simulink model "samePIDmodelworkingdecoupler_customsignal"  (R2018a)
settings: Solver=VariableStepAuto  StartTime=0.0  StopTime=100  RelTol=1e-3
undefined symbols (not defined in the file): sigbuilder_block
libraries: simulink x2
settings Model: Creator=40292302  LastModifiedBy=40292302

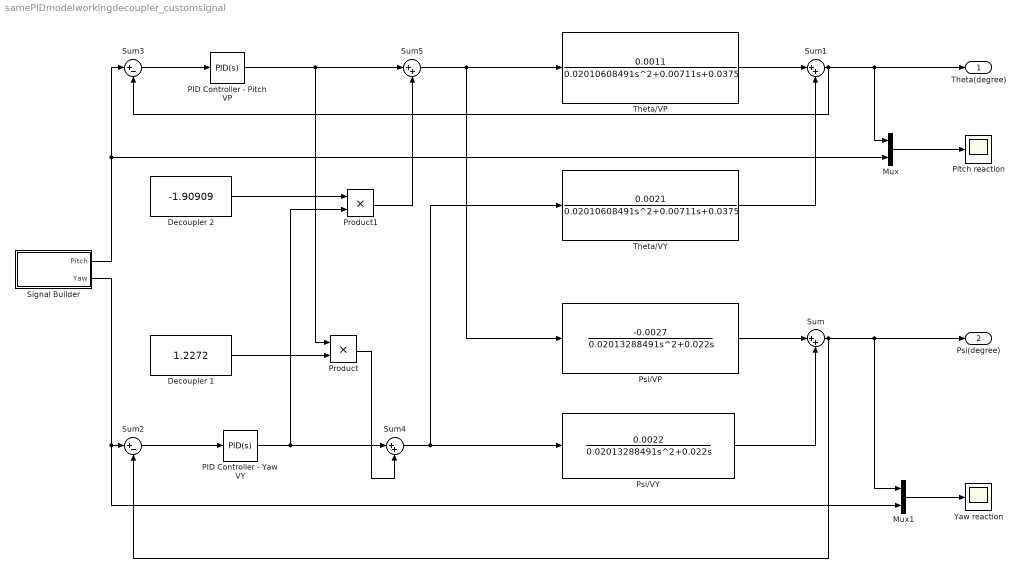
== system samePIDmodelworkingdecoupler_customsignal ==
  Decoupler 1 : Constant  Value=1.2272
  Decoupler 2 : Constant  Value=-1.90909
  Mux : Mux  Inputs=2
  Mux1 : Mux  Inputs=2
  PID Controller - Pitch VP : simulink/Continuous/PID Controller  Controller=PID  TimeDomain=Continuous-time  SampleTime=-1  IntegratorMethod=Forward Euler  FilterMethod=Forward Euler  Form=Parallel  UseFilter=on  ControllerParametersSource=internal  P=6813.01742872752  I=13170.6613633077  D=853.093750479044  N=251.511422827374  InitialConditionSource=internal  InitialConditionForIntegrator=0  InitialConditionForFilter=0  ExternalReset=none  LimitOutput=off  UpperSaturationLimit=inf  LowerSaturationLimit=-inf  LinearizeAsGain=on  AntiWindupMode=none  Kb=1  TrackingMode=off  Kt=1  PParamMin=[]  PParamMax=[]  IParamMin=[]  IParamMax=[]  DParamMin=[]  DParamMax=[]  NParamMin=[]  NParamMax=[]  KbParamMin=[]  KbParamMax=[]  KtParamMin=[]  KtParamMax=[]  POutMin=[]  POutMax=[]  IOutMin=[]  IOutMax=[]  DOutMin=[]  DOutMax=[]  NOutMin=[]  NOutMax=[]  KbOutMin=[]  KbOutMax=[]  KtOutMin=[]  KtOutMax=[]  IntegratorOutMin=[]  IntegratorOutMax=[]  FilterOutMin=[]  FilterOutMax=[]  SumOutMin=[]  SumOutMax=[]  SumI1OutMin=[]  SumI1OutMax=[]  SumI2OutMin=[]  SumI2OutMax=[]  SumI3OutMin=[]  SumI3OutMax=[]  SumDOutMin=[]  SumDOutMax=[]  SaturationOutMin=[]  SaturationOutMax=[]  IntegratorContinuousStateAttributes=''  IntegratorStateMustResolveToSignalObject=off  IntegratorRTWStateStorageClass=Auto  FilterContinuousStateAttributes=''  FilterStateMustResolveToSignalObject=off  FilterRTWStateStorageClass=Auto  DifferentiatorICPrevScaledInput=0  DifferentiatorOutMin=[]  DifferentiatorOutMax=[]  FilterDiffOutCoefMin=[]  FilterDiffOutCoefMax=[]  SumDenOutMin=[]  SumDenOutMax=[]  SumNumOutMin=[]  SumNumOutMax=[]  ReciprocalOutMin=[]  ReciprocalOutMax=[]  DivideOutMin=[]  DivideOutMax=[]  TunerSelectOption=Transfer Function Based (PID Tuner App)
  PID Controller - Yaw VY : simulink/Continuous/PID Controller  Controller=PID  TimeDomain=Continuous-time  SampleTime=-1  IntegratorMethod=Forward Euler  FilterMethod=Forward Euler  Form=Parallel  UseFilter=on  ControllerParametersSource=internal  P=185.640953081057  I=165.263118768111  D=51.5096134368126  N=207.04851488926  InitialConditionSource=internal  InitialConditionForIntegrator=0  InitialConditionForFilter=0  ExternalReset=none  LimitOutput=off  UpperSaturationLimit=inf  LowerSaturationLimit=-inf  LinearizeAsGain=on  AntiWindupMode=none  Kb=1  TrackingMode=off  Kt=1  PParamMin=[]  PParamMax=[]  IParamMin=[]  IParamMax=[]  DParamMin=[]  DParamMax=[]  NParamMin=[]  NParamMax=[]  KbParamMin=[]  KbParamMax=[]  KtParamMin=[]  KtParamMax=[]  POutMin=[]  POutMax=[]  IOutMin=[]  IOutMax=[]  DOutMin=[]  DOutMax=[]  NOutMin=[]  NOutMax=[]  KbOutMin=[]  KbOutMax=[]  KtOutMin=[]  KtOutMax=[]  IntegratorOutMin=[]  IntegratorOutMax=[]  FilterOutMin=[]  FilterOutMax=[]  SumOutMin=[]  SumOutMax=[]  SumI1OutMin=[]  SumI1OutMax=[]  SumI2OutMin=[]  SumI2OutMax=[]  SumI3OutMin=[]  SumI3OutMax=[]  SumDOutMin=[]  SumDOutMax=[]  SaturationOutMin=[]  SaturationOutMax=[]  IntegratorContinuousStateAttributes=''  IntegratorStateMustResolveToSignalObject=off  IntegratorRTWStateStorageClass=Auto  FilterContinuousStateAttributes=''  FilterStateMustResolveToSignalObject=off  FilterRTWStateStorageClass=Auto  DifferentiatorICPrevScaledInput=0  DifferentiatorOutMin=[]  DifferentiatorOutMax=[]  FilterDiffOutCoefMin=[]  FilterDiffOutCoefMax=[]  SumDenOutMin=[]  SumDenOutMax=[]  SumNumOutMin=[]  SumNumOutMax=[]  ReciprocalOutMin=[]  ReciprocalOutMax=[]  DivideOutMin=[]  DivideOutMax=[]  TunerSelectOption=Transfer Function Based (PID Tuner App)
  Pitch reaction : Scope
  Product : Product
  Product1 : Product
  Psi/VP : TransferFcn  Numerator=[-0.0027]  Denominator=[0.02013288491 0.022 0]
  Psi/VY : TransferFcn  Numerator=[0.0022]  Denominator=[0.02013288491 0.022 0]
  Signal Builder : Subsystem  Tag=STV Subsys  LoadFcn=sigbuilder_block('load');  StartFcn=sigbuilder_block('start');  StopFcn=sigbuilder_block('stop');  ClipboardFcn=sigbuilder_block('clipboard');  mask(Sigbuilder block){tuvar=[0:10]}
      mask help: Simulink:masks:SigbuilderBlock_MD
      mask init:
      | if ~strcmp(get_param(bdroot(gcbh),'SimulationStatus'),'stopped') tuvar = sigbuilder_block('maskInit'); end
      settings: CopyFcn=sigbuilder_block('copy');  DeleteFcn=sigbuilder_block('delete');  ModelCloseFcn=sigbuilder_block('modelClose');  PreSaveFcn=sigbuilder_block('preSave');  PauseFcn=sigbuilder_block('pause');  ContinueFcn=sigbuilder_block('continue');  NameChangeFcn=sigbuilder_block('namechange');  OpenFcn=sigbuilder_block('open',[408.75 -243.75 936 363.75 ]);  CloseFcn=sigbuilder_block('close');
      mask Display: plot(0, 0, 100, 100,[2, 2, 32, 32, 2], [68, 8, 8, 68, 68],[32, 2], [38, 38], [32, 19, 2],[53, 60, 44], [32, 17, 17, 2],[16, 16, 31, 31]);txt = getActiveGroup(gcbh);text(2, 100, txt,'verticalAlignment', 'top');
  Sum{,1,4..5} (4 alike) : Sum  Inputs=|++
  Sum2 : Sum  Inputs=|+-
  Sum3 : Sum  Inputs=|+-
  Theta/VP : TransferFcn  Numerator=[0.0011]  Denominator=[0.02010608491 0.00711 0.0375]
  Theta/VY : TransferFcn  Numerator=[0.0021]  Denominator=[0.02010608491 0.00711 0.0375]
  Yaw reaction : Scope
  Theta(degree) : Outport
  Psi(degree) : Outport  Port=2
  wires:
  Sum1/1 -> Theta(degree)/1, Mux/1, Sum3/2
  Theta/VP/1 -> Sum1/1
  Theta/VY/1 -> Sum1/2
  Psi/VP/1 -> Sum/1
  Psi/VY/1 -> Sum/2
  Mux/1 -> Pitch reaction/1
  Mux1/1 -> Yaw reaction/1
  Sum2/1 -> PID Controller - Yaw VY/1
  Sum/1 -> Psi(degree)/1, Mux1/1, Sum2/2
  Signal Builder/1(Pitch) -> Sum3/1, Mux/2
  Signal Builder/2(Yaw) -> Mux1/2, Sum2/1
  PID Controller - Pitch VP/1 -> Sum5/1, Product/1
  Sum3/1 -> PID Controller - Pitch VP/1
  PID Controller - Yaw VY/1 -> Sum4/1, Product1/2
  Sum4/1 -> Theta/VY/1, Psi/VY/1
  Product/1 -> Sum4/2
  Decoupler 1/1 -> Product/2
  Sum5/1 -> Psi/VP/1, Theta/VP/1
  Product1/1 -> Sum5/2
  Decoupler 2/1 -> Product1/1

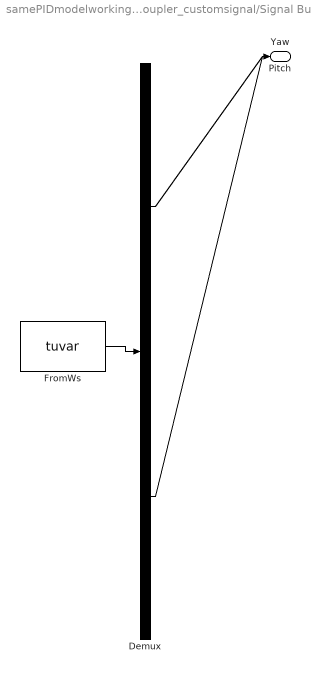
== system samePIDmodelworkingdecoupler_customsignal/Signal Builder ==
  Demux : Demux  Tag=STV Demux  Outputs=2
  FromWs : FromWorkspace  Tag=STV FromWs  VariableName=tuvar  SampleTime=0
      SigBuilderData=|
      | common.afterFinalStr = 'Extrapolate'
      | common.sampleTime = 0
      | dataSet.timeRange = [0 100]
      | dataSet.name = 'Group 1'
      | sbobj.Groups.Name = 'Group 1'
      | sbobj.Groups.Signals(1).Name = 'Pitch'
      | sbobj.Groups.Signals(1).XData = [0 10 20 30 30 40 40 50 60 60 70 70 100]
      | sbobj.Groups.Signals(1).YData = [0 0 0 0 15 15 -15 -15 -15 15 15 0 0]
      | sbobj.Groups.Signals(2).Name = 'Yaw'
      | sbobj.Groups.Signals(2).XData = [0 10 10 20 20 30 30 40 50 50 60 60 70 70 100]
      | sbobj.Groups.Signals(2).YData = [0 0 30 30 -30 -30 0 0 0 -30 -30 30 30 0 0]
      | sbobj.Groups.TimeRange = [0 100]
  Pitch : Outport  Tag=STV Outport
  Yaw : Outport  Tag=STV Outport  Port=2
  wires:
  FromWs/1 -> Demux/1
  Demux/1 -> Pitch/1
  Demux/2 -> Yaw/1
